simulink model "SCR_SiLS_R4_D102_test1"  (R2023a)
settings: Solver=VariableStepAuto  StartTime=0.0  StopTime=T_sim_end  RelTol=1e-3
model workspace (MAT data in the model file):
  ConnVar : object (value not decoded)
libraries: M1SWBlocks x4
(part 2 of 2)

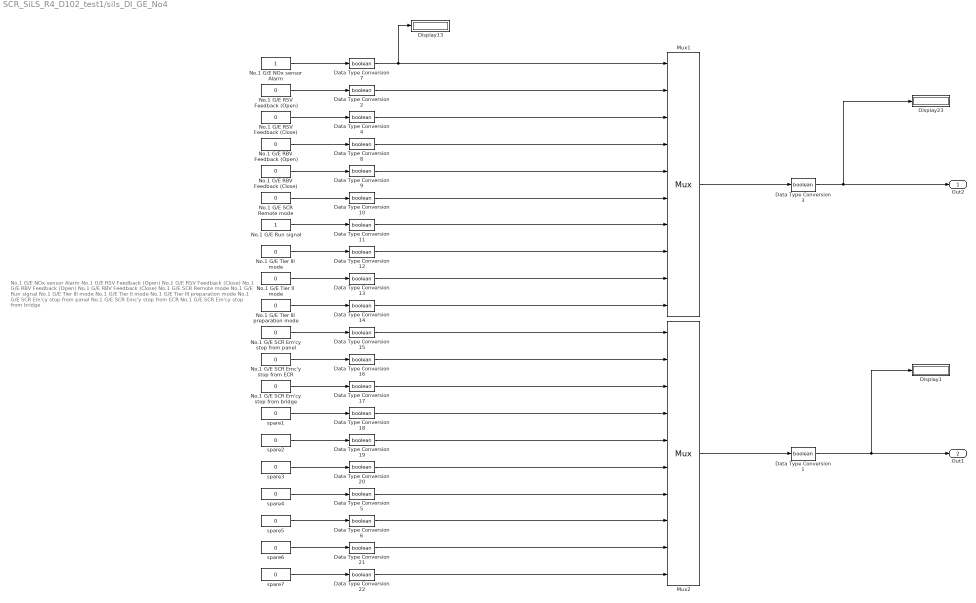
== system SCR_SiLS_R4_D102_test1/sils_DI_GE_No4 ==
  note: No.1 G/E NOx sensor Alarm
      |
      | No.1 G/E RSV Feedback (Open)
      |
      | No.1 G/E RSV Feedback (Close)
      |
      | No.1 G/E RBV Feedback (Open)
      |
      | No.1 G/E RBV Feedback (Close)
      |
      | No.1 G/E SCR Remote mode
      |
      | No.1 G/E Run signal
      |
      | No.1 G/E Tier III mode
      |
      | No.1 G/E Tier II mode
      |
      | No.1 G/E Tier III preparation mode
      |
      | No.1 G/E SCR Em'cy stop from panel
      |
      | No.1 G/E SCR Emc'y stop from ECR
      |
      | No.1 G/E SCR Em'cy stop from bridge
  Data Type Conversion{1..22} (22 alike) : DataTypeConversion  OutDataTypeStr=boolean  SaturateOnIntegerOverflow=off  RndMeth=Floor
  Display1 : Display
  Display13 : Display
  Display23 : Display
  Mux1 : Mux  Inputs=10
  Mux2 : Mux  Inputs=10
  No.1 G/E NOx sensor Alarm : Constant
  No.1 G/E RBV Feedback (Close) : Constant  Value=0
  No.1 G/E RBV Feedback (Open) : Constant  Value=0
  No.1 G/E RSV Feedback (Close) : Constant  Value=0
  No.1 G/E RSV Feedback (Open) : Constant  Value=0
  No.1 G/E Run signal : Constant
  No.1 G/E SCR Em'cy stop from bridge : Constant  Value=0
  No.1 G/E SCR Em'cy stop from panel : Constant  Value=0
  No.1 G/E SCR Emc'y stop from ECR : Constant  Value=0
  No.1 G/E SCR Remote mode : Constant  Value=0
  No.1 G/E Tier II mode : Constant  Value=0
  No.1 G/E Tier III mode : Constant  Value=0
  No.1 G/E Tier III preparation mode : Constant  Value=0
  spare{1..7} (7 alike) : Constant  Value=0
  Out2 : Outport
  Out1 : Outport  Port=2
  wires:
  No.1 G/E NOx sensor Alarm/1 -> Data Type Conversion7/1
  Data Type Conversion7/1 -> Display13/1, Mux1/1
  Data Type Conversion3/1 -> Out2/1, Display23/1
  Mux1/1 -> Data Type Conversion3/1
  No.1 G/E RSV Feedback (Open)/1 -> Data Type Conversion2/1
  No.1 G/E RSV Feedback (Close)/1 -> Data Type Conversion4/1
  No.1 G/E RBV Feedback (Open)/1 -> Data Type Conversion8/1
  No.1 G/E RBV Feedback (Close)/1 -> Data Type Conversion9/1
  No.1 G/E SCR Remote mode/1 -> Data Type Conversion10/1
  No.1 G/E Run signal/1 -> Data Type Conversion11/1
  No.1 G/E Tier III mode/1 -> Data Type Conversion12/1
  No.1 G/E Tier II mode/1 -> Data Type Conversion13/1
  No.1 G/E Tier III preparation mode/1 -> Data Type Conversion14/1
  No.1 G/E SCR Em'cy stop from panel/1 -> Data Type Conversion15/1
  No.1 G/E SCR Emc'y stop from ECR/1 -> Data Type Conversion16/1
  No.1 G/E SCR Em'cy stop from bridge/1 -> Data Type Conversion17/1
  spare1/1 -> Data Type Conversion18/1
  spare2/1 -> Data Type Conversion19/1
  spare3/1 -> Data Type Conversion20/1
  Data Type Conversion2/1 -> Mux1/2
  Data Type Conversion4/1 -> Mux1/3
  Data Type Conversion8/1 -> Mux1/4
  Data Type Conversion9/1 -> Mux1/5
  Data Type Conversion10/1 -> Mux1/6
  Data Type Conversion11/1 -> Mux1/7
  Data Type Conversion12/1 -> Mux1/8
  Data Type Conversion13/1 -> Mux1/9
  Data Type Conversion14/1 -> Mux1/10
  Data Type Conversion15/1 -> Mux2/1
  Data Type Conversion16/1 -> Mux2/2
  Data Type Conversion17/1 -> Mux2/3
  Data Type Conversion18/1 -> Mux2/4
  Data Type Conversion19/1 -> Mux2/5
  Data Type Conversion20/1 -> Mux2/6
  Data Type Conversion1/1 -> Out1/1, Display1/1
  Mux2/1 -> Data Type Conversion1/1
  spare4/1 -> Data Type Conversion5/1
  spare5/1 -> Data Type Conversion6/1
  Data Type Conversion5/1 -> Mux2/7
  Data Type Conversion6/1 -> Mux2/8
  spare6/1 -> Data Type Conversion21/1
  spare7/1 -> Data Type Conversion22/1
  Data Type Conversion21/1 -> Mux2/9
  Data Type Conversion22/1 -> Mux2/10

== system SCR_SiLS_R4_D102_test1/sils_DO_Comm ==
  note: DO output
      | Alarm Buzzer
      |
      | G/E SCR common alarm lamp
      |
      | No.1 Urea supply pump Start
      |
      | No.1 Urea supply pump Stop
      |
      | No.2 Urea supply pump Start
      |
      | No.2 Urea supply pump Stop
      |
      | G/E SCR common Alarm
      |
      | G/E SCR Em'cy Stopped
      |
      | No.1 Urea supply pump Running
      |
      | No.2 Urea supply pump Running
      |
      | No.1 G/E SCR Common Alarm lamp
      |
      | No.2 G/E SCR Common Alarm lamp
      |
      | No.3 G/E SCR Common Alarm lamp
      |
      | No.4 G/E SCR Common Alarm lamp
      |
      | ​
      |
      | ​
  In1 : Inport
  In2 : Inport  Port=2
  Demux1 : Demux  Outputs=10
  Demux2 : Demux  Outputs=10
  Display{14..17,24,30..40} (16 alike) : Display
  wires:
  Demux1/7 -> Display31/1  "G/E SCR common Alarm"
  Demux1/8 -> Display32/1  "G/E SCR Em'cy Stopped"
  Demux1/9 -> Display33/1  "No.1 Urea supply pump Running"
  In1/1 -> Demux1/1
  Demux1/1 -> Display24/1  "Alarm Buzzer"
  Demux1/3 -> Display15/1  "No.1 Urea supply pump Start"
  Demux1/5 -> Display17/1  "No.2 Urea supply pump Start"
  Demux1/4 -> Display16/1  "No.1 Urea supply pump Stop"
  Demux1/6 -> Display30/1  "No.2 Urea supply pump Stop"
  Demux2/6 -> Display40/1
  Demux1/2 -> Display14/1  "G/E SCR common alarm lamp"
  Demux2/5 -> Display39/1
  Demux1/10 -> Display34/1  "No.2 Urea supply pump Running"
  Demux2/3 -> Display37/1  "No.3 G/E SCR Common Alarm lamp"
  Demux2/4 -> Display38/1  "No.4 G/E SCR Common Alarm lamp"
  Demux2/2 -> Display36/1  "No.2 G/E SCR Common Alarm lamp"
  Demux2/1 -> Display35/1  "No.1 G/E SCR Common Alarm lamp"
  In2/1 -> Demux2/1

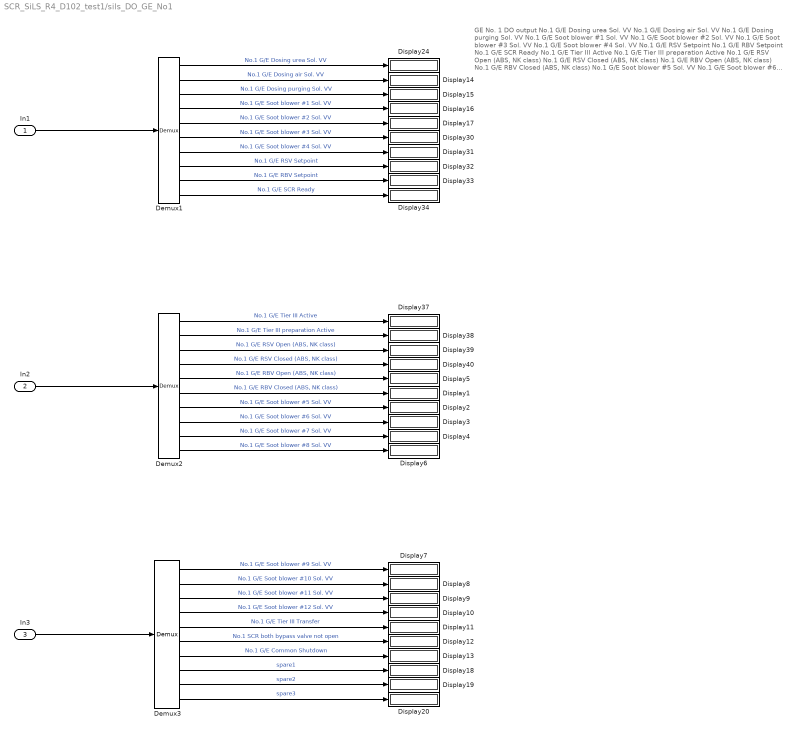
== system SCR_SiLS_R4_D102_test1/sils_DO_GE_No1 ==
  note: GE No. 1 DO output
      |
      | No.1 G/E Dosing urea Sol. VV
      |
      | No.1 G/E Dosing air Sol. VV
      |
      | No.1 G/E Dosing purging Sol. VV
      |
      | No.1 G/E Soot blower #1 Sol. VV
      |
      | No.1 G/E Soot blower #2 Sol. VV
      |
      | No.1 G/E Soot blower #3 Sol. VV
      |
      | No.1 G/E Soot blower #4 Sol. VV
      |
      | No.1 G/E RSV Setpoint
      |
      | No.1 G/E RBV Setpoint
      |
      | No.1 G/E SCR Ready
      |
      | No.1 G/E Tier III Active
      |
      | No.1 G/E Tier III preparation Active
      |
      | No.1 G/E RSV Open (ABS, NK class)
      |
      | No.1 G/E RSV Closed (ABS, NK class)
      |
      | No.1 G/E RBV Open (ABS, NK class)
      |
      | No.1 G/E RBV Closed (ABS, NK class)
      |
      | No.1 G/E Soot blower #5 Sol. VV
      |
      | No.1 G/E Soot blower #6 Sol. VV
      |
      | No.1 G/E Soot blower #7 Sol. VV
      |
      | No.1 G/E Soot blower #8 Sol. VV
      |
      | No.1 G/E Soot blower #9 Sol. VV
      |
      | No.1 G/E Soot blower #10 Sol. VV
      |
      | No.1 G/E Soot blower #11 Sol. VV
      |
      | No.1 G/E Soot blower #12 Sol. VV
      |
      | No.1 G/E Tier III Transfer
      |
      | No.1 SCR both bypass valve not open
      |
      | No.# G/E Common Shutdown
  In1 : Inport
  In2 : Inport  Port=2
  In3 : Inport  Port=3
  Demux1 : Demux  Outputs=10
  Demux2 : Demux  Outputs=10
  Demux3 : Demux  Outputs=10
  Display{1..20,24,30..34,37..40} (30 alike) : Display
  wires:
  Demux1/7 -> Display31/1  "No.1 G/E Soot blower #4 Sol. VV"
  Demux1/8 -> Display32/1  "No.1 G/E RSV Setpoint"
  Demux1/9 -> Display33/1  "No.1 G/E RBV Setpoint"
  In1/1 -> Demux1/1
  Demux1/1 -> Display24/1  "No.1 G/E Dosing urea Sol. VV"
  Demux1/3 -> Display15/1  "No.1 G/E Dosing purging Sol. VV"
  Demux1/5 -> Display17/1  "No.1 G/E Soot blower #2 Sol. VV"
  Demux1/4 -> Display16/1  "No.1 G/E Soot blower #1 Sol. VV"
  Demux1/6 -> Display30/1  "No.1 G/E Soot blower #3 Sol. VV"
  Demux2/6 -> Display1/1  "No.1 G/E RBV Closed (ABS, NK class)"
  Demux1/2 -> Display14/1  "No.1 G/E Dosing air Sol. VV"
  Demux2/5 -> Display5/1  "No.1 G/E RBV Open (ABS, NK class)"
  Demux1/10 -> Display34/1  "No.1 G/E SCR Ready"
  Demux2/3 -> Display39/1  "No.1 G/E RSV Open (ABS, NK class)"
  Demux2/4 -> Display40/1  "No.1 G/E RSV Closed (ABS, NK class)"
  Demux2/2 -> Display38/1  "No.1 G/E Tier III preparation Active"
  Demux2/1 -> Display37/1  "No.1 G/E Tier III Active"
  Demux2/7 -> Display2/1  "No.1 G/E Soot blower #5 Sol. VV"
  Demux3/9 -> Display19/1  "spare2"
  Demux3/6 -> Display12/1  "No.1 SCR both bypass valve not open"
  Demux3/7 -> Display13/1  "No.1 G/E Common Shutdown"
  Demux2/8 -> Display3/1  "No.1 G/E Soot blower #6 Sol. VV"
  Demux3/1 -> Display7/1  "No.1 G/E Soot blower #9 Sol. VV"
  Demux3/10 -> Display20/1  "spare3"
  In2/1 -> Demux2/1
  Demux3/4 -> Display10/1  "No.1 G/E Soot blower #12 Sol. VV"
  Demux2/10 -> Display6/1  "No.1 G/E Soot blower #8 Sol. VV"
  Demux3/2 -> Display8/1  "No.1 G/E Soot blower #10 Sol. VV"
  Demux3/8 -> Display18/1  "spare1"
  Demux3/5 -> Display11/1  "No.1 G/E Tier III Transfer"
  Demux2/9 -> Display4/1  "No.1 G/E Soot blower #7 Sol. VV"
  Demux3/3 -> Display9/1  "No.1 G/E Soot blower #11 Sol. VV"
  In3/1 -> Demux3/1

== system SCR_SiLS_R4_D102_test1/sils_DO_GE_No2 ==
  note: GE No. 1 DO output
      |
      | No.1 G/E Dosing urea Sol. VV
      |
      | No.1 G/E Dosing air Sol. VV
      |
      | No.1 G/E Dosing purging Sol. VV
      |
      | No.1 G/E Soot blower #1 Sol. VV
      |
      | No.1 G/E Soot blower #2 Sol. VV
      |
      | No.1 G/E Soot blower #3 Sol. VV
      |
      | No.1 G/E Soot blower #4 Sol. VV
      |
      | No.1 G/E RSV Setpoint
      |
      | No.1 G/E RBV Setpoint
      |
      | No.1 G/E SCR Ready
      |
      | No.1 G/E Tier III Active
      |
      | No.1 G/E Tier III preparation Active
      |
      | No.1 G/E RSV Open (ABS, NK class)
      |
      | No.1 G/E RSV Closed (ABS, NK class)
      |
      | No.1 G/E RBV Open (ABS, NK class)
      |
      | No.1 G/E RBV Closed (ABS, NK class)
      |
      | No.1 G/E Soot blower #5 Sol. VV
      |
      | No.1 G/E Soot blower #6 Sol. VV
      |
      | No.1 G/E Soot blower #7 Sol. VV
      |
      | No.1 G/E Soot blower #8 Sol. VV
      |
      | No.1 G/E Soot blower #9 Sol. VV
      |
      | No.1 G/E Soot blower #10 Sol. VV
      |
      | No.1 G/E Soot blower #11 Sol. VV
      |
      | No.1 G/E Soot blower #12 Sol. VV
      |
      | No.1 G/E Tier III Transfer
      |
      | No.1 SCR both bypass valve not open
      |
      | No.# G/E Common Shutdown
  In1 : Inport
  In2 : Inport  Port=2
  In3 : Inport  Port=3
  Demux1 : Demux  Outputs=10
  Demux2 : Demux  Outputs=10
  Demux3 : Demux  Outputs=10
  Display{1..20,24,30..34,37..40} (30 alike) : Display
  wires:
  Demux1/7 -> Display31/1  "No.1 G/E Soot blower #4 Sol. VV"
  Demux1/8 -> Display32/1  "No.1 G/E RSV Setpoint"
  Demux1/9 -> Display33/1  "No.1 G/E RBV Setpoint"
  In1/1 -> Demux1/1
  Demux1/1 -> Display24/1  "No.1 G/E Dosing urea Sol. VV"
  Demux1/3 -> Display15/1  "No.1 G/E Dosing purging Sol. VV"
  Demux1/5 -> Display17/1  "No.1 G/E Soot blower #2 Sol. VV"
  Demux1/4 -> Display16/1  "No.1 G/E Soot blower #1 Sol. VV"
  Demux1/6 -> Display30/1  "No.1 G/E Soot blower #3 Sol. VV"
  Demux2/6 -> Display1/1  "No.1 G/E RBV Closed (ABS, NK class)"
  Demux1/2 -> Display14/1  "No.1 G/E Dosing air Sol. VV"
  Demux2/5 -> Display5/1  "No.1 G/E RBV Open (ABS, NK class)"
  Demux1/10 -> Display34/1  "No.1 G/E SCR Ready"
  Demux2/3 -> Display39/1  "No.1 G/E RSV Open (ABS, NK class)"
  Demux2/4 -> Display40/1  "No.1 G/E RSV Closed (ABS, NK class)"
  Demux2/2 -> Display38/1  "No.1 G/E Tier III preparation Active"
  Demux2/1 -> Display37/1  "No.1 G/E Tier III Active"
  Demux2/7 -> Display2/1  "No.1 G/E Soot blower #5 Sol. VV"
  Demux3/9 -> Display19/1  "spare2"
  Demux3/6 -> Display12/1  "No.1 SCR both bypass valve not open"
  Demux3/7 -> Display13/1  "No.1 G/E Common Shutdown"
  Demux2/8 -> Display3/1  "No.1 G/E Soot blower #6 Sol. VV"
  Demux3/1 -> Display7/1  "No.1 G/E Soot blower #9 Sol. VV"
  Demux3/10 -> Display20/1  "spare3"
  In2/1 -> Demux2/1
  Demux3/4 -> Display10/1  "No.1 G/E Soot blower #12 Sol. VV"
  Demux2/10 -> Display6/1  "No.1 G/E Soot blower #8 Sol. VV"
  Demux3/2 -> Display8/1  "No.1 G/E Soot blower #10 Sol. VV"
  Demux3/8 -> Display18/1  "spare1"
  Demux3/5 -> Display11/1  "No.1 G/E Tier III Transfer"
  Demux2/9 -> Display4/1  "No.1 G/E Soot blower #7 Sol. VV"
  Demux3/3 -> Display9/1  "No.1 G/E Soot blower #11 Sol. VV"
  In3/1 -> Demux3/1

== system SCR_SiLS_R4_D102_test1/sils_DO_GE_No3 ==
  note: GE No. 1 DO output
      |
      | No.1 G/E Dosing urea Sol. VV
      |
      | No.1 G/E Dosing air Sol. VV
      |
      | No.1 G/E Dosing purging Sol. VV
      |
      | No.1 G/E Soot blower #1 Sol. VV
      |
      | No.1 G/E Soot blower #2 Sol. VV
      |
      | No.1 G/E Soot blower #3 Sol. VV
      |
      | No.1 G/E Soot blower #4 Sol. VV
      |
      | No.1 G/E RSV Setpoint
      |
      | No.1 G/E RBV Setpoint
      |
      | No.1 G/E SCR Ready
      |
      | No.1 G/E Tier III Active
      |
      | No.1 G/E Tier III preparation Active
      |
      | No.1 G/E RSV Open (ABS, NK class)
      |
      | No.1 G/E RSV Closed (ABS, NK class)
      |
      | No.1 G/E RBV Open (ABS, NK class)
      |
      | No.1 G/E RBV Closed (ABS, NK class)
      |
      | No.1 G/E Soot blower #5 Sol. VV
      |
      | No.1 G/E Soot blower #6 Sol. VV
      |
      | No.1 G/E Soot blower #7 Sol. VV
      |
      | No.1 G/E Soot blower #8 Sol. VV
      |
      | No.1 G/E Soot blower #9 Sol. VV
      |
      | No.1 G/E Soot blower #10 Sol. VV
      |
      | No.1 G/E Soot blower #11 Sol. VV
      |
      | No.1 G/E Soot blower #12 Sol. VV
      |
      | No.1 G/E Tier III Transfer
      |
      | No.1 SCR both bypass valve not open
      |
      | No.# G/E Common Shutdown
  In1 : Inport
  In2 : Inport  Port=2
  In3 : Inport  Port=3
  Demux1 : Demux  Outputs=10
  Demux2 : Demux  Outputs=10
  Demux3 : Demux  Outputs=10
  Display{1..20,24,30..34,37..40} (30 alike) : Display
  wires:
  Demux1/7 -> Display31/1  "No.1 G/E Soot blower #4 Sol. VV"
  Demux1/8 -> Display32/1  "No.1 G/E RSV Setpoint"
  Demux1/9 -> Display33/1  "No.1 G/E RBV Setpoint"
  In1/1 -> Demux1/1
  Demux1/1 -> Display24/1  "No.1 G/E Dosing urea Sol. VV"
  Demux1/3 -> Display15/1  "No.1 G/E Dosing purging Sol. VV"
  Demux1/5 -> Display17/1  "No.1 G/E Soot blower #2 Sol. VV"
  Demux1/4 -> Display16/1  "No.1 G/E Soot blower #1 Sol. VV"
  Demux1/6 -> Display30/1  "No.1 G/E Soot blower #3 Sol. VV"
  Demux2/6 -> Display1/1  "No.1 G/E RBV Closed (ABS, NK class)"
  Demux1/2 -> Display14/1  "No.1 G/E Dosing air Sol. VV"
  Demux2/5 -> Display5/1  "No.1 G/E RBV Open (ABS, NK class)"
  Demux1/10 -> Display34/1  "No.1 G/E SCR Ready"
  Demux2/3 -> Display39/1  "No.1 G/E RSV Open (ABS, NK class)"
  Demux2/4 -> Display40/1  "No.1 G/E RSV Closed (ABS, NK class)"
  Demux2/2 -> Display38/1  "No.1 G/E Tier III preparation Active"
  Demux2/1 -> Display37/1  "No.1 G/E Tier III Active"
  Demux2/7 -> Display2/1  "No.1 G/E Soot blower #5 Sol. VV"
  Demux3/9 -> Display19/1  "spare2"
  Demux3/6 -> Display12/1  "No.1 SCR both bypass valve not open"
  Demux3/7 -> Display13/1  "No.1 G/E Common Shutdown"
  Demux2/8 -> Display3/1  "No.1 G/E Soot blower #6 Sol. VV"
  Demux3/1 -> Display7/1  "No.1 G/E Soot blower #9 Sol. VV"
  Demux3/10 -> Display20/1  "spare3"
  In2/1 -> Demux2/1
  Demux3/4 -> Display10/1  "No.1 G/E Soot blower #12 Sol. VV"
  Demux2/10 -> Display6/1  "No.1 G/E Soot blower #8 Sol. VV"
  Demux3/2 -> Display8/1  "No.1 G/E Soot blower #10 Sol. VV"
  Demux3/8 -> Display18/1  "spare1"
  Demux3/5 -> Display11/1  "No.1 G/E Tier III Transfer"
  Demux2/9 -> Display4/1  "No.1 G/E Soot blower #7 Sol. VV"
  Demux3/3 -> Display9/1  "No.1 G/E Soot blower #11 Sol. VV"
  In3/1 -> Demux3/1

== system SCR_SiLS_R4_D102_test1/sils_DO_GE_No4 ==
  note: GE No. 1 DO output
      |
      | No.1 G/E Dosing urea Sol. VV
      |
      | No.1 G/E Dosing air Sol. VV
      |
      | No.1 G/E Dosing purging Sol. VV
      |
      | No.1 G/E Soot blower #1 Sol. VV
      |
      | No.1 G/E Soot blower #2 Sol. VV
      |
      | No.1 G/E Soot blower #3 Sol. VV
      |
      | No.1 G/E Soot blower #4 Sol. VV
      |
      | No.1 G/E RSV Setpoint
      |
      | No.1 G/E RBV Setpoint
      |
      | No.1 G/E SCR Ready
      |
      | No.1 G/E Tier III Active
      |
      | No.1 G/E Tier III preparation Active
      |
      | No.1 G/E RSV Open (ABS, NK class)
      |
      | No.1 G/E RSV Closed (ABS, NK class)
      |
      | No.1 G/E RBV Open (ABS, NK class)
      |
      | No.1 G/E RBV Closed (ABS, NK class)
      |
      | No.1 G/E Soot blower #5 Sol. VV
      |
      | No.1 G/E Soot blower #6 Sol. VV
      |
      | No.1 G/E Soot blower #7 Sol. VV
      |
      | No.1 G/E Soot blower #8 Sol. VV
      |
      | No.1 G/E Soot blower #9 Sol. VV
      |
      | No.1 G/E Soot blower #10 Sol. VV
      |
      | No.1 G/E Soot blower #11 Sol. VV
      |
      | No.1 G/E Soot blower #12 Sol. VV
      |
      | No.1 G/E Tier III Transfer
      |
      | No.1 SCR both bypass valve not open
      |
      | No.# G/E Common Shutdown
  In1 : Inport
  In2 : Inport  Port=2
  In3 : Inport  Port=3
  Demux1 : Demux  Outputs=10
  Demux2 : Demux  Outputs=10
  Demux3 : Demux  Outputs=10
  Display{1..20,24,30..34,37..40} (30 alike) : Display
  wires:
  Demux1/7 -> Display31/1  "No.1 G/E Soot blower #4 Sol. VV"
  Demux1/8 -> Display32/1  "No.1 G/E RSV Setpoint"
  Demux1/9 -> Display33/1  "No.1 G/E RBV Setpoint"
  In1/1 -> Demux1/1
  Demux1/1 -> Display24/1  "No.1 G/E Dosing urea Sol. VV"
  Demux1/3 -> Display15/1  "No.1 G/E Dosing purging Sol. VV"
  Demux1/5 -> Display17/1  "No.1 G/E Soot blower #2 Sol. VV"
  Demux1/4 -> Display16/1  "No.1 G/E Soot blower #1 Sol. VV"
  Demux1/6 -> Display30/1  "No.1 G/E Soot blower #3 Sol. VV"
  Demux2/6 -> Display1/1  "No.1 G/E RBV Closed (ABS, NK class)"
  Demux1/2 -> Display14/1  "No.1 G/E Dosing air Sol. VV"
  Demux2/5 -> Display5/1  "No.1 G/E RBV Open (ABS, NK class)"
  Demux1/10 -> Display34/1  "No.1 G/E SCR Ready"
  Demux2/3 -> Display39/1  "No.1 G/E RSV Open (ABS, NK class)"
  Demux2/4 -> Display40/1  "No.1 G/E RSV Closed (ABS, NK class)"
  Demux2/2 -> Display38/1  "No.1 G/E Tier III preparation Active"
  Demux2/1 -> Display37/1  "No.1 G/E Tier III Active"
  Demux2/7 -> Display2/1  "No.1 G/E Soot blower #5 Sol. VV"
  Demux3/9 -> Display19/1  "spare2"
  Demux3/6 -> Display12/1  "No.1 SCR both bypass valve not open"
  Demux3/7 -> Display13/1  "No.1 G/E Common Shutdown"
  Demux2/8 -> Display3/1  "No.1 G/E Soot blower #6 Sol. VV"
  Demux3/1 -> Display7/1  "No.1 G/E Soot blower #9 Sol. VV"
  Demux3/10 -> Display20/1  "spare3"
  In2/1 -> Demux2/1
  Demux3/4 -> Display10/1  "No.1 G/E Soot blower #12 Sol. VV"
  Demux2/10 -> Display6/1  "No.1 G/E Soot blower #8 Sol. VV"
  Demux3/2 -> Display8/1  "No.1 G/E Soot blower #10 Sol. VV"
  Demux3/8 -> Display18/1  "spare1"
  Demux3/5 -> Display11/1  "No.1 G/E Tier III Transfer"
  Demux2/9 -> Display4/1  "No.1 G/E Soot blower #7 Sol. VV"
  Demux3/3 -> Display9/1  "No.1 G/E Soot blower #11 Sol. VV"
  In3/1 -> Demux3/1
